simulink model "controller"  (R2020a)
settings: Solver=ode45  StartTime=0.0  StopTime=120  RelTol=1e-3
model workspace (MAT data in the model file):
  b = 50
  ki = 4.5
  kp = 22
  m = 1000
  u = 500
settings Model: Creator=Admin  LastModifiedBy=Admin

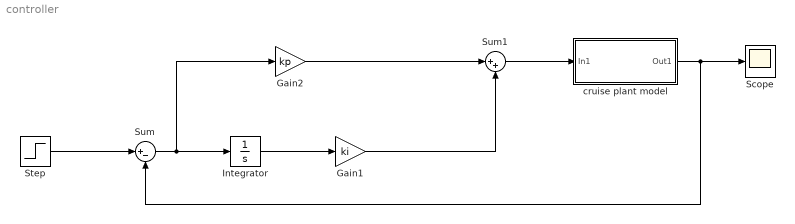
== system controller ==
  Gain1 : Gain  Gain=ki
  Gain2 : Gain  Gain=kp
  Integrator : Integrator
  Scope : Scope
  Step : Step  Time=0  After=u  SampleTime=0
  Sum : Sum  Inputs=|+-
  Sum1 : Sum  Inputs=|++
  cruise plant model : Subsystem
  wires:
  Step/1 -> Sum/1
  Sum/1 -> Gain2/1, Integrator/1
  Integrator/1 -> Gain1/1
  Gain1/1 -> Sum1/2
  Gain2/1 -> Sum1/1
  Sum1/1 -> cruise plant model/1(In1)
  cruise plant model/1(Out1) -> Sum/2, Scope/1

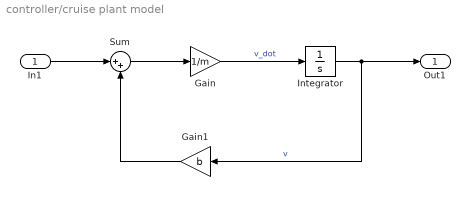
== system controller/cruise plant model ==
  In1 : Inport
  Gain : Gain  Gain=1/m
  Gain1 : Gain  Gain=b
  Integrator : Integrator
  Sum : Sum  Inputs=|++
  Out1 : Outport
  wires:
  Integrator/1 -> Gain1/1, Out1/1  "v"
  In1/1 -> Sum/1
  Sum/1 -> Gain/1
  Gain/1 -> Integrator/1  "v_dot"
  Gain1/1 -> Sum/2
